simulink subsystem "rss_PhCurrCalc"  (R2023a)
settings: Solver=VariableStepAuto  StartTime=0.0  StopTime=10.0  RelTol=1e-3
undefined symbols (not defined in the file): Cdbl_iPhCurrMaxVal
libraries: lib_magnitude_calculator x1, lib_moving_average_filter x1
settings Model: DefaultTestHarness=rss_LineCurrentCalculation_thu  Creator=CAV2OFO  LastModifiedBy=xiaoqiang.yuan
settings OptimizationCC: ReuseModelBlockBuffer=off

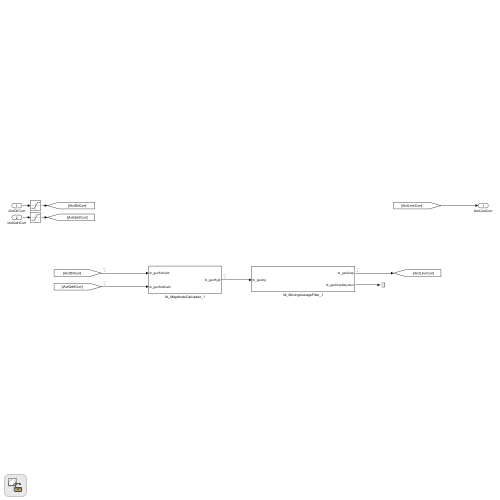
[thumbnail: Simulink's stored preview of the top-level diagram]
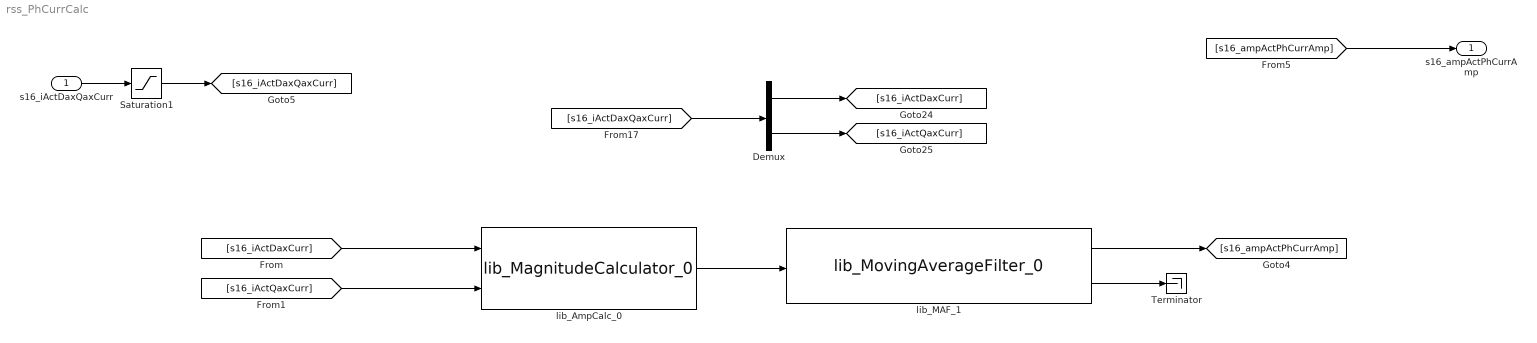
== system rss_PhCurrCalc ==
  s16_iActDaxQaxCurr : Inport  OutDataTypeStr=dt_Standardize_s16p15b0
  Demux : Demux  Outputs=2
  Saturation1 : Saturate  UpperLimit=Cdbl_iPhCurrMaxVal  LowerLimit=-Cdbl_iPhCurrMaxVal
  Terminator : Terminator
  lib_AmpCalc_0 : lib_magnitude_calculator/lib_MagnitudeCalculator_0  lb_parLktSize=512  lb_parOutpDataType=dt_Standardize_s16p15b0
  lib_MAF_1 : lib_moving_average_filter/lib_MovingAverageFilter_0  lb_parSampNum=Cdbl_numPhCurrMAFSmpNum  lb_parInpSmtnDataType=fixdt(1,32,2^-19,0)
  s16_ampActPhCurrAmp : Outport  OutDataTypeStr=dt_Standardize_s16p15b0
  wires:
  lib_MAF_1/1 -> [s16_ampActPhCurrAmp]
  lib_AmpCalc_0/1 -> lib_MAF_1/1
  [s16_iActDaxCurr] -> lib_AmpCalc_0/1
  [s16_iActQaxCurr] -> lib_AmpCalc_0/2
  [s16_ampActPhCurrAmp] -> s16_ampActPhCurrAmp/1
  lib_MAF_1/2 -> Terminator/1
  s16_iActDaxQaxCurr/1 -> Saturation1/1
  Saturation1/1 -> [s16_iActDaxQaxCurr]
  [s16_iActDaxQaxCurr] -> Demux/1
  Demux/2 -> [s16_iActQaxCurr]
  Demux/1 -> [s16_iActDaxCurr]
